simulink library "ifo"  (Simulink 8.2)
settings: Solver=ode45  StartTime=0.0  StopTime=10.0  RelTol=1e-3
undefined symbols (not defined in the file or in its folder): ENUM_EPSADASABREASON_NO_DRIVING_INTERRUPTION, ENUM_GEARPOSN_1ST, ENUM_GEARPOSN_2ND, ENUM_GEARPOSN_3RD, ENUM_GEARPOSN_4TH, ENUM_GEARPOSN_5TH, ENUM_GEARPOSN_6TH, ENUM_LFCSTATE_AUTOSTEERING, ENUM_LFCSTATE_DEGRADED, ENUM_SHIFTLEVER_D, ENUM_SHIFTLEVER_D2, ENUM_SHIFTLEVER_D3, FALSE, KAPP_VehicleWidth_m, KIFO_C1Max4Act_rad, KIFO_C2Max4Act_rat, KIFO_C2Max4Disable_rat, KIFO_C2Max4DisableThr_s, KIFO_DriverStrFightConfirmTime_s, KIFO_DriverStrFightResetTime_s, KIFO_DriverStrFightSetTime_s, KIFO_DriverStrFightThres_Nm, KIFO_DriverStrFightThresHys_Nm, KIFO_DriverStrSoftConfirmTime_s, KIFO_DriverStrSoftResetTime_s, KIFO_DriverStrSoftSetTime_s, KIFO_DriverStrSoftThres_Nm, KIFO_DriverStrStrongConfirmTime_s, KIFO_DriverStrStrongResetTime_s, KIFO_DriverStrStrongSetTime_s, KIFO_DriverStrStrongThres_Nm, KIFO_DriverStrStrongThresHys_Nm, KIFO_Lane4ActThr_s, KIFO_LaneWidthLowThr_m, KIFO_LaneWidthUpThr_m, KIFO_LFCVehSpdMaxLimition_kph, KIFO_LFCVehSpdMimLimition_kph, KIFO_LKAMaxActSpeed_kph, KIFO_LKAMaxDeactSpeed_kph, KIFO_LKAMinActSpeed_kph, KIFO_LKAMinDeactSpeed_kph, KIFO_TLCTriggerThrHysis_s, KIFO_TurnSignalSwOFFTime_s, MIFO_TLCThr4LKA_s, TRUE
libraries: hcu_lib x41, simulink x11, hmi x1, gaps x1, ttc x1, sft x1, veh x1
(part 1 of 2)
settings Model: Creator=xsellart  LastModifiedBy=13192

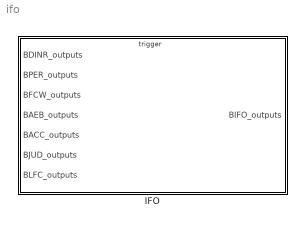
== system ifo ==
  IFO : Subsystem

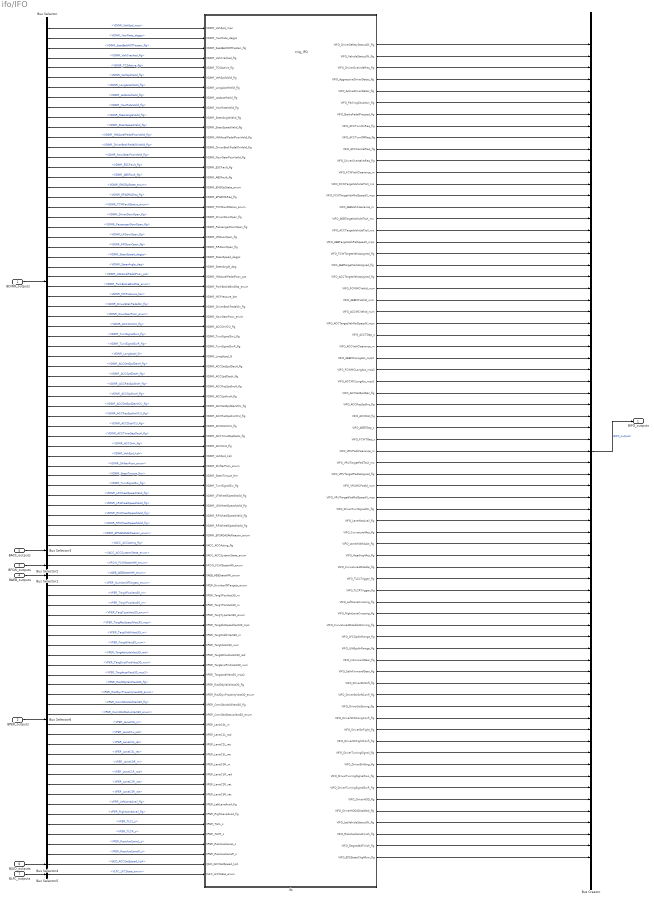
== system ifo/IFO ==
  BDINR_outputs : Inport  OutDataTypeStr=Bus: BDINR_outputs
  BPER_outputs : Inport  Port=2  OutDataTypeStr=Bus: BPER_outputs
  BFCW_outputs : Inport  Port=3  OutDataTypeStr=Bus: BFCW_outputs
  BAEB_outputs : Inport  Port=4  OutDataTypeStr=Bus: BAEB_outputs
  BACC_outputs : Inport  Port=5  OutDataTypeStr=Bus: BACC_outputs
  BJUD_outputs : Inport  Port=6  OutDataTypeStr=Bus: BJUD_outputs
  BLFC_outputs : Inport  Port=7  OutDataTypeStr=Bus: BLFC_outputs
  trig_IFO : TriggerPort  TriggerType=function-call
      settings: AttributesFormatString=State = %<StatesWhenEnabling>
  Bus Creator : BusCreator  Inputs=71  OutDataTypeStr=Bus: BIFO_outputs
  Bus Selector : BusSelector  OutputSignals=VDINR_VehSpd_mps,VDINR_YawRate_degps,VDINR_SeatBeltNOTFasten_flg,VDINR_VehCrashed_flg,VDINR_TCSActive_flg,VDINR_VehSpdValid_flg,VDINR_LongAccelValid_flg,VDINR_LatAccelValid_flg,VDINR_YawRateValid_flg,VDINR_SteerAngleValid_flg,VDINR_SteerSpeedValid_flg,VDINR_HWAccelPedalPosnValid_flg,VDINR_DriverBrakPedalOnValid_flg,VDINR_NowGearPosnValid_flg,VDINR_ESCFault_flg,VDINR_ABSFault_flg,VDINR_EMSOpState_enum,VDINR_EPASMILReq_flg,VDINR_TCMFaultStatus_enum,VDINR_DriverDoorOpen_flg,VDINR_PassengerDoorOpen_flg,VDINR_LRDoorOpen_flg,VDINR_RRDoorOpen_flg,VDINR_SteerSpeed_degps,VDINR_SteerAngle_deg,VDINR_HWAccelPedalPosn_pct,VDINR_ParkBrakeBindSta_enum,VDINR_MCPressure_bar,VDINR_DriverBrakPedalOn_flg,VDINR_NowGearPosn_enum,VDINR_ACCOnVCU_flg,VDINR_TurnSignalSwL_flg,VDINR_TurnSignalSwR_flg,VDINR_LongAccel_G,VDINR_ACCSetSpdDecH_flg,VDINR_ACCSpdDecH_flg,VDINR_ACCResSpdIncH_flg,VDINR_ACCSpdIncH_flg,VDINR_ACCSetSpdDecVCU_flg,VDINR_ACCResSpdIncVCU_flg,VDINR_ACCDistVCU_flg,VDINR_ACCTimeGapDecH_flg,VDINR_ACCOnH_flg,VDINR_VehSpd_kph,VDINR_ShifterPosn_enum,VDINR_SteerTorque_Nm,VDINR_TurnSignalSw_flg,VDINR_LFWheelSpeedValid_flg,VDINR_LRWheelSpeedValid_flg,VDINR_RFWheelSpeedValid_flg,VDINR_RRWheelSpeedValid_flg,VDINR_EPSADASAbReason_enum
  Bus Selector1 : BusSelector  OutputSignals=VAEB_AEBStateHMI_enum
  Bus Selector2 : BusSelector  OutputSignals=VFCW_FCWStateHMI_enum
  Bus Selector3 : BusSelector  OutputSignals=VACC_ACCActing_flg,VACC_ACCSystemState_enum
  Bus Selector4 : BusSelector  OutputSignals=VJUD_ACCSetSpeed_kph
  Bus Selector5 : BusSelector  OutputSignals=VLFC_LFCState_enum
  Bus Selector6 : BusSelector  OutputSignals=VPER_NumberOfTargets_enum,VPER_TargXPosVect30_m,VPER_TargYPosVect30_m,VPER_TargTypeVect30_enum,VPER_TargAbsSpeedVect30_mps,VPER_TargWidthVect30_m,VPER_TargIdVect30_num,VPER_TargAttitudeVect30_rad,VPER_TargExistProbVect30_num,VPER_TargAccelVect30_mps2,VPER_RadObjValidVect30_flg,VPER_RadDynPropertyVect30_enum,VPER_CamObsValidVect30_flg,VPER_CamObsStatusVect30_enum,VPER_LaneC0L_m,VPER_LaneC1L_rad,VPER_LaneC2L_rat,VPER_LaneC3L_rat,VPER_LaneC0R_m,VPER_LaneC1R_rad,VPER_LaneC2R_rat,VPER_LaneC3R_rat,VPER_LeftLaneAvail_flg,VPER_RightLaneAvail_flg,VPER_TLCL_s,VPER_TLCR_s,VPER_ResidualLaneL_s,VPER_ResidualLaneR_s
  ifo : Subsystem
  BIFO_outputs : Outport  OutDataTypeStr=Bus: BIFO_outputs
  wires:
  BDINR_outputs/1 -> Bus Selector/1
  BFCW_outputs/1 -> Bus Selector2/1
  BPER_outputs/1 -> Bus Selector6/1
  Bus Creator/1 -> BIFO_outputs/1  "BIFO_outputs"
  BAEB_outputs/1 -> Bus Selector1/1
  Bus Selector/19 -> ifo/19(VDINR_TCMFaultStatus_enum)  "<VDINR_TCMFaultStatus_enum>"
  Bus Selector/21 -> ifo/21(VDINR_PassengerDoorOpen_flg)  "<VDINR_PassengerDoorOpen_flg>"
  Bus Selector/13 -> ifo/13(VDINR_DriverBrakPedalOnValid_flg)  "<VDINR_DriverBrakPedalOnValid_flg>"
  Bus Selector/11 -> ifo/11(VDINR_SteerSpeedValid_flg)  "<VDINR_SteerSpeedValid_flg>"
  Bus Selector/17 -> ifo/17(VDINR_EMSOpState_enum)  "<VDINR_EMSOpState_enum>"
  Bus Selector/12 -> ifo/12(VDINR_HWAccelPedalPosnValid_flg)  "<VDINR_HWAccelPedalPosnValid_flg>"
  Bus Selector/14 -> ifo/14(VDINR_NowGearPosnValid_flg)  "<VDINR_NowGearPosnValid_flg>"
  Bus Selector/18 -> ifo/18(VDINR_EPASMILReq_flg)  "<VDINR_EPASMILReq_flg>"
  Bus Selector/16 -> ifo/16(VDINR_ABSFault_flg)  "<VDINR_ABSFault_flg>"
  Bus Selector/8 -> ifo/8(VDINR_LatAccelValid_flg)  "<VDINR_LatAccelValid_flg>"
  Bus Selector/20 -> ifo/20(VDINR_DriverDoorOpen_flg)  "<VDINR_DriverDoorOpen_flg>"
  Bus Selector/9 -> ifo/9(VDINR_YawRateValid_flg)  "<VDINR_YawRateValid_flg>"
  Bus Selector/15 -> ifo/15(VDINR_ESCFault_flg)  "<VDINR_ESCFault_flg>"
  Bus Selector/10 -> ifo/10(VDINR_SteerAngleValid_flg)  "<VDINR_SteerAngleValid_flg>"
  Bus Selector/22 -> ifo/22(VDINR_LRDoorOpen_flg)  "<VDINR_LRDoorOpen_flg>"
  Bus Selector/23 -> ifo/23(VDINR_RRDoorOpen_flg)  "<VDINR_RRDoorOpen_flg>"
  Bus Selector/3 -> ifo/3(VDINR_SeatBeltNOTFasten_flg)  "<VDINR_SeatBeltNOTFasten_flg>"
  Bus Selector/6 -> ifo/6(VDINR_VehSpdValid_flg)  "<VDINR_VehSpdValid_flg>"
  Bus Selector/24 -> ifo/24(VDINR_SteerSpeed_degps)  "<VDINR_SteerSpeed_degps>"
  Bus Selector/2 -> ifo/2(VDINR_YawRate_degps)  "<VDINR_YawRate_degps>"
  Bus Selector/4 -> ifo/4(VDINR_VehCrashed_flg)  "<VDINR_VehCrashed_flg>"
  Bus Selector/1 -> ifo/1(VDINR_VehSpd_mps)  "<VDINR_VehSpd_mps>"
  Bus Selector/7 -> ifo/7(VDINR_LongAccelValid_flg)  "<VDINR_LongAccelValid_flg>"
  Bus Selector/5 -> ifo/5(VDINR_TCSActive_flg)  "<VDINR_TCSActive_flg>"
  Bus Selector/30 -> ifo/30(VDINR_NowGearPosn_enum)  "<VDINR_NowGearPosn_enum>"
  Bus Selector/29 -> ifo/29(VDINR_DriverBrakPedalOn_flg)  "<VDINR_DriverBrakPedalOn_flg>"
  Bus Selector/28 -> ifo/28(VDINR_MCPressure_bar)  "<VDINR_MCPressure_bar>"
  Bus Selector/27 -> ifo/27(VDINR_ParkBrakeBindSta_enum)  "<VDINR_ParkBrakeBindSta_enum>"
  Bus Selector/26 -> ifo/26(VDINR_HWAccelPedalPosn_pct)  "<VDINR_HWAccelPedalPosn_pct>"
  Bus Selector/25 -> ifo/25(VDINR_SteerAngle_deg)  "<VDINR_SteerAngle_deg>"
  BACC_outputs/1 -> Bus Selector3/1
  Bus Selector1/1 -> ifo/56(VAEB_AEBStateHMI_enum)  "<VAEB_AEBStateHMI_enum>"
  Bus Selector2/1 -> ifo/55(VFCW_FCWStateHMI_enum)  "<VFCW_FCWStateHMI_enum>"
  Bus Selector3/1 -> ifo/53(VACC_ACCActing_flg)  "<VACC_ACCActing_flg>"
  Bus Selector3/2 -> ifo/54(VACC_ACCSystemState_enum)  "<VACC_ACCSystemState_enum>"
  Bus Selector/32 -> ifo/32(VDINR_TurnSignalSwL_flg)  "<VDINR_TurnSignalSwL_flg>"
  BJUD_outputs/1 -> Bus Selector4/1
  Bus Selector4/1 -> ifo/85(VJUD_ACCSetSpeed_kph)  "<VJUD_ACCSetSpeed_kph>"
  Bus Selector/31 -> ifo/31(VDINR_ACCOnVCU_flg)  "<VDINR_ACCOnVCU_flg>"
  Bus Selector/34 -> ifo/34(VDINR_LongAccel_G)  "<VDINR_LongAccel_G>"
  Bus Selector/35 -> ifo/35(VDINR_ACCSetSpdDecH_flg)  "<VDINR_ACCSetSpdDecH_flg>"
  Bus Selector/36 -> ifo/36(VDINR_ACCSpdDecH_flg)  "<VDINR_ACCSpdDecH_flg>"
  Bus Selector/37 -> ifo/37(VDINR_ACCResSpdIncH_flg)  "<VDINR_ACCResSpdIncH_flg>"
  Bus Selector/38 -> ifo/38(VDINR_ACCSpdIncH_flg)  "<VDINR_ACCSpdIncH_flg>"
  Bus Selector/40 -> ifo/40(VDINR_ACCResSpdIncVCU_flg)  "<VDINR_ACCResSpdIncVCU_flg>"
  Bus Selector/39 -> ifo/39(VDINR_ACCSetSpdDecVCU_flg)  "<VDINR_ACCSetSpdDecVCU_flg>"
  Bus Selector/43 -> ifo/43(VDINR_ACCOnH_flg)  "<VDINR_ACCOnH_flg>"
  Bus Selector/42 -> ifo/42(VDINR_ACCTimeGapDecH_flg)  "<VDINR_ACCTimeGapDecH_flg>"
  Bus Selector/41 -> ifo/41(VDINR_ACCDistVCU_flg)  "<VDINR_ACCDistVCU_flg>"
  Bus Selector/33 -> ifo/33(VDINR_TurnSignalSwR_flg)  "<VDINR_TurnSignalSwR_flg>"
  Bus Selector/44 -> ifo/44(VDINR_VehSpd_kph)  "<VDINR_VehSpd_kph>"
  Bus Selector/45 -> ifo/45(VDINR_ShifterPosn_enum)  "<VDINR_ShifterPosn_enum>"
  Bus Selector/48 -> ifo/48(VDINR_LFWheelSpeedValid_flg)  "<VDINR_LFWheelSpeedValid_flg>"
  Bus Selector/47 -> ifo/47(VDINR_TurnSignalSw_flg)  "<VDINR_TurnSignalSw_flg>"
  Bus Selector/46 -> ifo/46(VDINR_SteerTorque_Nm)  "<VDINR_SteerTorque_Nm>"
  Bus Selector/49 -> ifo/49(VDINR_LRWheelSpeedValid_flg)  "<VDINR_LRWheelSpeedValid_flg>"
  Bus Selector/51 -> ifo/51(VDINR_RRWheelSpeedValid_flg)  "<VDINR_RRWheelSpeedValid_flg>"
  Bus Selector/50 -> ifo/50(VDINR_RFWheelSpeedValid_flg)  "<VDINR_RFWheelSpeedValid_flg>"
  Bus Selector6/8 -> ifo/64(VPER_TargAttitudeVect30_rad)  "<VPER_TargAttitudeVect30_rad>"
  Bus Selector6/9 -> ifo/65(VPER_TargExisProbVect30_num)  "<VPER_TargExistProbVect30_num>"
  Bus Selector6/7 -> ifo/63(VPER_TargIdVect30_num)  "<VPER_TargIdVect30_num>"
  Bus Selector6/6 -> ifo/62(VPER_TargWidthVect30_m)  "<VPER_TargWidthVect30_m>"
  Bus Selector6/10 -> ifo/66(VPER_TargAccelVect30_mps2)  "<VPER_TargAccelVect30_mps2>"
  Bus Selector6/5 -> ifo/61(VPER_TargAbsSpeedVect30_mps)  "<VPER_TargAbsSpeedVect30_mps>"
  Bus Selector6/11 -> ifo/67(VPER_RadObjValidVect30_flg)  "<VPER_RadObjValidVect30_flg>"
  Bus Selector6/4 -> ifo/60(VPER_TargTypeVect30_enum)  "<VPER_TargTypeVect30_enum>"
  Bus Selector6/12 -> ifo/68(VPER_RadDynPropertyVect30_enum)  "<VPER_RadDynPropertyVect30_enum>"
  Bus Selector6/3 -> ifo/59(VPER_TargYPosVect30_m)  "<VPER_TargYPosVect30_m>"
  Bus Selector6/13 -> ifo/69(VPER_CamObsValidVect30_flg)  "<VPER_CamObsValidVect30_flg>"
  Bus Selector6/2 -> ifo/58(VPER_TargXPosVect30_m)  "<VPER_TargXPosVect30_m>"
  Bus Selector6/14 -> ifo/70(VPER_CamObsStatusVect30_enum)  "<VPER_CamObsStatusVect30_enum>"
  Bus Selector6/1 -> ifo/57(VPER_NumberOfTargets_enum)  "<VPER_NumberOfTargets_enum>"
  Bus Selector6/15 -> ifo/71(VPER_LaneC0L_m)  "<VPER_LaneC0L_m>"
  Bus Selector6/16 -> ifo/72(VPER_LaneC1L_rad)  "<VPER_LaneC1L_rad>"
  Bus Selector6/17 -> ifo/73(VPER_LaneC2L_rat)  "<VPER_LaneC2L_rat>"
  Bus Selector6/18 -> ifo/74(VPER_LaneC3L_rat)  "<VPER_LaneC3L_rat>"
  Bus Selector6/19 -> ifo/75(VPER_LaneC0R_m)  "<VPER_LaneC0R_m>"
  Bus Selector6/20 -> ifo/76(VPER_LaneC1R_rad)  "<VPER_LaneC1R_rad>"
  Bus Selector6/21 -> ifo/77(VPER_LaneC2R_rat)  "<VPER_LaneC2R_rat>"
  Bus Selector6/22 -> ifo/78(VPER_LaneC3R_rat)  "<VPER_LaneC3R_rat>"
  Bus Selector6/23 -> ifo/79(VPER_LeftLaneAvail_fig)  "<VPER_LeftLaneAvail_flg>"
  Bus Selector6/24 -> ifo/80(VPER_RightLaneAvail_fig)  "<VPER_RightLaneAvail_flg>"
  Bus Selector6/25 -> ifo/81(VPER_TLCL_s)  "<VPER_TLCL_s>"
  Bus Selector6/26 -> ifo/82(VPER_TLCR_s)  "<VPER_TLCR_s>"
  Bus Selector6/27 -> ifo/83(VPER_ResidualLaneL_s)  "<VPER_ResidualLaneL_s>"
  Bus Selector6/28 -> ifo/84(VPER_ResidualLaneR_s)  "<VPER_ResidualLaneR_s>"
  ifo/17(VIFO_ACCTargetVehicleTtcX_ms) -> Bus Creator/17
  ifo/18(VIFO_AEBTargetVehRelSpeedX_mps) -> Bus Creator/18
  ifo/16(VIFO_AEBTargetVehicleTtcX_ms) -> Bus Creator/16
  ifo/15(VIFO_AEBVehClearance_m) -> Bus Creator/15
  ifo/19(VIFO_FCWTargetVehAssigned_flg) -> Bus Creator/19
  ifo/14(VIFO_FCWTargetVehRelSpeedX_mps) -> Bus Creator/14
  ifo/20(VIFO_AEBTargetVehAssigned_flg) -> Bus Creator/20
  ifo/13(VIFO_FCWTargetVehicleTtcX_ms) -> Bus Creator/13
  ifo/21(VIFO_ACCTargetVehAssigned_flg) -> Bus Creator/21
  ifo/12(VIFO_FCWVehClearance_m) -> Bus Creator/12
  ifo/22(VIFO_FCWMCVehId_num) -> Bus Creator/22
  ifo/11(VIFO_DriverOvertakeReq_flg) -> Bus Creator/11
  ifo/23(VIFO_AEBMCVehId_num) -> Bus Creator/23
  ifo/24(VIFO_ACCMCVehId_num) -> Bus Creator/24
  ifo/10(VIFO_ACCCancelReq_flg) -> Bus Creator/10
  ifo/9(VIFO_ACCTurnOffReq_flg) -> Bus Creator/9
  ifo/25(VIFO_ACCTargetVehRelSpeedX_mps) -> Bus Creator/25
  ifo/8(VIFO_ACCTurnOnReq_flg) -> Bus Creator/8
  ifo/26(VIFO_ACCTGap_s) -> Bus Creator/26
  ifo/7(VIFO_BrakePedalPressed_flg) -> Bus Creator/7
  ifo/27(VIFO_ACCVehClearance_m) -> Bus Creator/27
  ifo/28(VIFO_AEBMCLongAcc_mps2) -> Bus Creator/28
  ifo/6(VIFO_ParkingSituation_flg) -> Bus Creator/6
  ifo/29(VIFO_FCWMCLongAcc_mps2) -> Bus Creator/29
  ifo/5(VIFO_ActiveDriverDetec_flg) -> Bus Creator/5
  ifo/4(VIFO_AggressiveDriverDetec_flg) -> Bus Creator/4
  ifo/30(VIFO_ACCMCLongAcc_mps2) -> Bus Creator/30
  ifo/3(VIFO_DriverOverrideReq_flg) -> Bus Creator/3
  ifo/31(VIFO_ACCSetSpdDec_flg) -> Bus Creator/31
  ifo/32(VIFO_ACCResSpdInc_flg) -> Bus Creator/32
  ifo/2(VIFO_VehicleStatusOk_flg) -> Bus Creator/2
  ifo/1(VIFO_DriverSafetyStatusOk_flg) -> Bus Creator/1
  ifo/33(VIFO_ACCDist_flg) -> Bus Creator/33
  ifo/34(VIFO_AEBTGap_s) -> Bus Creator/34
  ifo/35(VIFO_FCWTGap_s) -> Bus Creator/35
  ifo/36(VIFO_VRUPedClearance_m) -> Bus Creator/36
  ifo/37(VIFO_VRUTargetPedTtcX_ms) -> Bus Creator/37
  ifo/38(VIFO_VRUTargetPedAssigned_flg) -> Bus Creator/38
  ifo/39(VIFO_VRUMCPedId_num) -> Bus Creator/39
  ifo/40(VIFO_VRUTargetPedRelSpeedX_mps) -> Bus Creator/40
  ifo/41(VIFO_DriverTurnSignalOn_flg) -> Bus Creator/41
  ifo/42(VIFO_LaneNotAvail_flg) -> Bus Creator/42
  ifo/43(VIFO_Curvature4Act_flg) -> Bus Creator/43
  ifo/44(VIFO_LaneWidth4Act_flg) -> Bus Creator/44
  ifo/45(VIFO_Heading4Act_flg) -> Bus Creator/45
  ifo/46(VIFO_Curvature4Disable_flg) -> Bus Creator/46
  ifo/47(VIFO_TLCLTrigger_flg) -> Bus Creator/47
  ifo/48(VIFO_TLCRTrigger_flg) -> Bus Creator/48
  ifo/49(VIFO_LeftLaneCrossing_flg) -> Bus Creator/49
  ifo/50(VIFO_RightLaneCrossing_flg) -> Bus Creator/50
  ifo/51(VIFO_Curvature4DisableWarning_flg) -> Bus Creator/51
  ifo/52(VIFO_LFCSpdInRange_flg) -> Bus Creator/52
  ifo/53(VIFO_LKASpdInRange_flg) -> Bus Creator/53
  ifo/54(VIFO_InForwardGear_flg) -> Bus Creator/54
  ifo/55(VIFO_SelInForwardGear_flg) -> Bus Creator/55
  ifo/56(VIFO_DriverStrSoft_flg) -> Bus Creator/56
  ifo/57(VIFO_DriverStrSoftConfi_flg) -> Bus Creator/57
  ifo/58(VIFO_DriverStrStrong_flg) -> Bus Creator/58
  ifo/59(VIFO_DriverStrStrongConfi_flg) -> Bus Creator/59
  ifo/60(VIFO_DriverStrFight_flg) -> Bus Creator/60
  ifo/61(VIFO_DriverStrFightConfi_flg) -> Bus Creator/61
  ifo/62(VIFO_DriverTurningSignal_flg) -> Bus Creator/62
  ifo/63(VIFO_DriverShifting_flg) -> Bus Creator/63
  ifo/64(VIFO_DriverTurningSignalSwL_flg) -> Bus Creator/64
  ifo/65(VIFO_DriverTurningSignalSwR_flg) -> Bus Creator/65
  ifo/66(VIFO_DriverHOD_flg) -> Bus Creator/66
  ifo/67(VIFO_DriverHOD4Disabled_flg) -> Bus Creator/67
  ifo/68(VIFO_LatVehicleStatusOk_flg) -> Bus Creator/68
  ifo/69(VIFO_ResidualLaneFinish_flg) -> Bus Creator/69
  ifo/70(VIFO_DegradedFinish_flg) -> Bus Creator/70
  BLFC_outputs/1 -> Bus Selector5/1
  Bus Selector5/1 -> ifo/86(VLFC_LFCState_enum)  "<VLFC_LFCState_enum>"
  Bus Selector/52 -> ifo/52(VDINR_EPSADASAbReason_enum)  "<VDINR_EPSADASAbReason_enum>"
  ifo/71(VIFO_EPSStateChgAllow_flg) -> Bus Creator/71

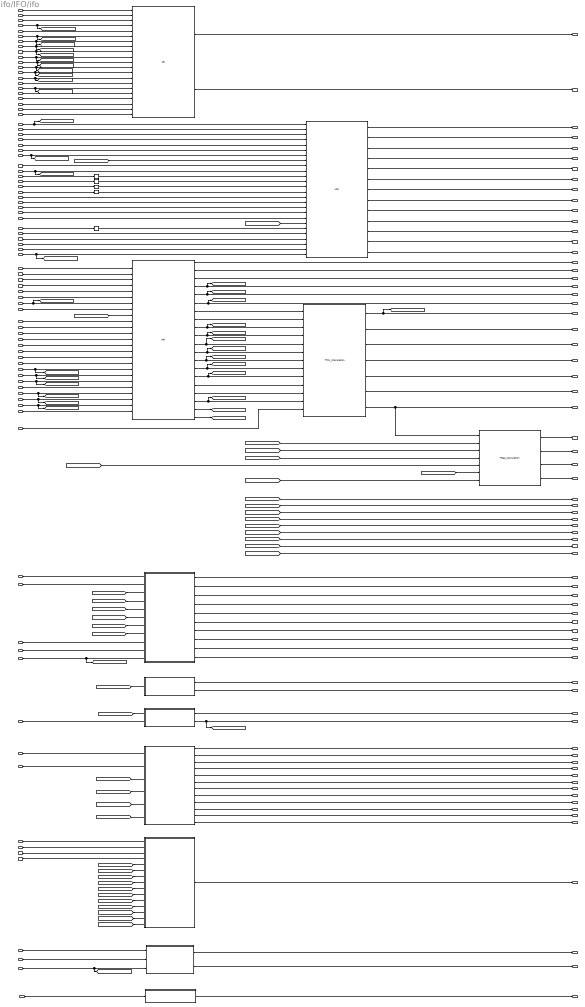
== system ifo/IFO/ifo ==
  VDINR_VehSpd_mps : Inport
  VDINR_YawRate_degps : Inport  Port=2
  VDINR_SeatBeltNOTFasten_flg : Inport  Port=3
  VDINR_VehCrashed_flg : Inport  Port=4
  VDINR_TCSActive_flg : Inport  Port=5
  VDINR_VehSpdValid_flg : Inport  Port=6
  VDINR_LongAccelValid_flg : Inport  Port=7
  VDINR_LatAccelValid_flg : Inport  Port=8
  VDINR_YawRateValid_flg : Inport  Port=9
  VDINR_SteerAngleValid_flg : Inport  Port=10
  VDINR_SteerSpeedValid_flg : Inport  Port=11
  VDINR_HWAccelPedalPosnValid_flg : Inport  Port=12
  VDINR_DriverBrakPedalOnValid_flg : Inport  Port=13
  VDINR_NowGearPosnValid_flg : Inport  Port=14
  VDINR_ESCFault_flg : Inport  Port=15
  VDINR_ABSFault_flg : Inport  Port=16
  VDINR_EMSOpState_enum : Inport  Port=17
  VDINR_EPASMILReq_flg : Inport  Port=18
  VDINR_TCMFaultStatus_enum : Inport  Port=19
  VDINR_DriverDoorOpen_flg : Inport  Port=20
  VDINR_PassengerDoorOpen_flg : Inport  Port=21
  VDINR_LRDoorOpen_flg : Inport  Port=22
  VDINR_RRDoorOpen_flg : Inport  Port=23
  VDINR_SteerSpeed_degps : Inport  Port=24
  VDINR_SteerAngle_deg : Inport  Port=25
  VDINR_HWAccelPedalPosn_pct : Inport  Port=26
  VDINR_ParkBrakeBindSta_enum : Inport  Port=27
  VDINR_MCPressure_bar : Inport  Port=28
  VDINR_DriverBrakPedalOn_flg : Inport  Port=29
  VDINR_NowGearPosn_enum : Inport  Port=30
  VDINR_ACCOnVCU_flg : Inport  Port=31
  VDINR_TurnSignalSwL_flg : Inport  Port=32
  VDINR_TurnSignalSwR_flg : Inport  Port=33
  VDINR_LongAccel_G : Inport  Port=34
  VDINR_ACCSetSpdDecH_flg : Inport  Port=35
  VDINR_ACCSpdDecH_flg : Inport  Port=36
  VDINR_ACCResSpdIncH_flg : Inport  Port=37
  VDINR_ACCSpdIncH_flg : Inport  Port=38
  VDINR_ACCSetSpdDecVCU_flg : Inport  Port=39
  VDINR_ACCResSpdIncVCU_flg : Inport  Port=40
  VDINR_ACCDistVCU_flg : Inport  Port=41
  VDINR_ACCTimeGapDecH_flg : Inport  Port=42
  VDINR_ACCOnH_flg : Inport  Port=43
  VDINR_VehSpd_kph : Inport  Port=44
  VDINR_ShifterPosn_enum : Inport  Port=45
  VDINR_SteerTorque_Nm : Inport  Port=46
  VDINR_TurnSignalSw_flg : Inport  Port=47
  VDINR_LFWheelSpeedValid_flg : Inport  Port=48
  VDINR_LRWheelSpeedValid_flg : Inport  Port=49
  VDINR_RFWheelSpeedValid_flg : Inport  Port=50
  VDINR_RRWheelSpeedValid_flg : Inport  Port=51
  VDINR_EPSADASAbReason_enum : Inport  Port=52
  VACC_ACCActing_flg : Inport  Port=53
  VACC_ACCSystemState_enum : Inport  Port=54
  VFCW_FCWStateHMI_enum : Inport  Port=55
  VAEB_AEBStateHMI_enum : Inport  Port=56
  VPER_NumberOfTargets_enum : Inport  Port=57
  VPER_TargXPosVect30_m : Inport  Port=58
  VPER_TargYPosVect30_m : Inport  Port=59
  VPER_TargTypeVect30_enum : Inport  Port=60
  VPER_TargAbsSpeedVect30_mps : Inport  Port=61
  VPER_TargWidthVect30_m : Inport  Port=62
  VPER_TargIdVect30_num : Inport  Port=63
  VPER_TargAttitudeVect30_rad : Inport  Port=64
  VPER_TargExisProbVect30_num : Inport  Port=65
  VPER_TargAccelVect30_mps2 : Inport  Port=66
  VPER_RadObjValidVect30_flg : Inport  Port=67
  VPER_RadDynPropertyVect30_enum : Inport  Port=68
  VPER_CamObsValidVect30_flg : Inport  Port=69
  VPER_CamObsStatusVect30_enum : Inport  Port=70
  VPER_LaneC0L_m : Inport  Port=71
  VPER_LaneC1L_rad : Inport  Port=72
  VPER_LaneC2L_rat : Inport  Port=73
  VPER_LaneC3L_rat : Inport  Port=74
  VPER_LaneC0R_m : Inport  Port=75
  VPER_LaneC1R_rad : Inport  Port=76
  VPER_LaneC2R_rat : Inport  Port=77
  VPER_LaneC3R_rat : Inport  Port=78
  VPER_LeftLaneAvail_fig : Inport  Port=79
  VPER_RightLaneAvail_fig : Inport  Port=80
  VPER_TLCL_s : Inport  Port=81
  VPER_TLCR_s : Inport  Port=82
  VPER_ResidualLaneL_s : Inport  Port=83
  VPER_ResidualLaneR_s : Inport  Port=84
  VJUD_ACCSetSpeed_kph : Inport  Port=85
  VLFC_LFCState_enum : Inport  Port=86
  Delay{,1..4} (5 alike) : Delay  DelayLength=1  InitialCondition=0
  DriverIntentDecision : Subsystem  TreatAsAtomicUnit=on
  EPSStatus : Subsystem  TreatAsAtomicUnit=on
  HMI : hmi/HMI
  InForwardGearDetection : Subsystem  TreatAsAtomicUnit=on
  LFCLaneWarning_Decision : Subsystem
  LaneInfo : Subsystem  TreatAsAtomicUnit=on
  SpdInRange : Subsystem  TreatAsAtomicUnit=on
  TGap_Calculation : gaps/TGap_Calculation
  TTCx_Calculation : ttc/TTCx_Calculation
  VehicleStatusForLateral : Subsystem  TreatAsAtomicUnit=on
  sft : sft/sft
  veh : veh/veh
  VIFO_DriverSafetyStatusOk_flg : Outport
  VIFO_VehicleStatusOk_flg : Outport  Port=2
  VIFO_DriverOverrideReq_flg : Outport  Port=3
  VIFO_AggressiveDriverDetec_flg : Outport  Port=4
  VIFO_ActiveDriverDetec_flg : Outport  Port=5
  VIFO_ParkingSituation_flg : Outport  Port=6
  VIFO_BrakePedalPressed_flg : Outport  Port=7
  VIFO_ACCTurnOnReq_flg : Outport  Port=8
  VIFO_ACCTurnOffReq_flg : Outport  Port=9
  VIFO_ACCCancelReq_flg : Outport  Port=10
  VIFO_DriverOvertakeReq_flg : Outport  Port=11
  VIFO_FCWVehClearance_m : Outport  Port=12
  VIFO_FCWTargetVehicleTtcX_ms : Outport  Port=13
  VIFO_FCWTargetVehRelSpeedX_mps : Outport  Port=14
  VIFO_AEBVehClearance_m : Outport  Port=15
  VIFO_AEBTargetVehicleTtcX_ms : Outport  Port=16
  VIFO_ACCTargetVehicleTtcX_ms : Outport  Port=17
  VIFO_AEBTargetVehRelSpeedX_mps : Outport  Port=18
  VIFO_FCWTargetVehAssigned_flg : Outport  Port=19
  VIFO_AEBTargetVehAssigned_flg : Outport  Port=20
  VIFO_ACCTargetVehAssigned_flg : Outport  Port=21
  VIFO_FCWMCVehId_num : Outport  Port=22
  VIFO_AEBMCVehId_num : Outport  Port=23
  VIFO_ACCMCVehId_num : Outport  Port=24
  VIFO_ACCTargetVehRelSpeedX_mps : Outport  Port=25
  VIFO_ACCTGap_s : Outport  Port=26
  VIFO_ACCVehClearance_m : Outport  Port=27
  VIFO_AEBMCLongAcc_mps2 : Outport  Port=28
  VIFO_FCWMCLongAcc_mps2 : Outport  Port=29
  VIFO_ACCMCLongAcc_mps2 : Outport  Port=30
  VIFO_ACCSetSpdDec_flg : Outport  Port=31
  VIFO_ACCResSpdInc_flg : Outport  Port=32
  VIFO_ACCDist_flg : Outport  Port=33
  VIFO_AEBTGap_s : Outport  Port=34
  VIFO_FCWTGap_s : Outport  Port=35
  VIFO_VRUPedClearance_m : Outport  Port=36
  VIFO_VRUTargetPedTtcX_ms : Outport  Port=37
  VIFO_VRUTargetPedAssigned_flg : Outport  Port=38
  VIFO_VRUMCPedId_num : Outport  Port=39
  VIFO_VRUTargetPedRelSpeedX_mps : Outport  Port=40
  VIFO_DriverTurnSignalOn_flg : Outport  Port=41
  VIFO_LaneNotAvail_flg : Outport  Port=42
  VIFO_Curvature4Act_flg : Outport  Port=43
  VIFO_LaneWidth4Act_flg : Outport  Port=44
  VIFO_Heading4Act_flg : Outport  Port=45
  VIFO_Curvature4Disable_flg : Outport  Port=46
  VIFO_TLCLTrigger_flg : Outport  Port=47
  VIFO_TLCRTrigger_flg : Outport  Port=48
  VIFO_LeftLaneCrossing_flg : Outport  Port=49
  VIFO_RightLaneCrossing_flg : Outport  Port=50
  VIFO_Curvature4DisableWarning_flg : Outport  Port=51
  VIFO_LFCSpdInRange_flg : Outport  Port=52
  VIFO_LKASpdInRange_flg : Outport  Port=53
  VIFO_InForwardGear_flg : Outport  Port=54
  VIFO_SelInForwardGear_flg : Outport  Port=55
  VIFO_DriverStrSoft_flg : Outport  Port=56
  VIFO_DriverStrSoftConfi_flg : Outport  Port=57
  VIFO_DriverStrStrong_flg : Outport  Port=58
  VIFO_DriverStrStrongConfi_flg : Outport  Port=59
  VIFO_DriverStrFight_flg : Outport  Port=60
  VIFO_DriverStrFightConfi_flg : Outport  Port=61
  VIFO_DriverTurningSignal_flg : Outport  Port=62
  VIFO_DriverShifting_flg : Outport  Port=63
  VIFO_DriverTurningSignalSwL_flg : Outport  Port=64
  VIFO_DriverTurningSignalSwR_flg : Outport  Port=65
  VIFO_DriverHOD_flg : Outport  Port=66
  VIFO_DriverHOD4Disabled_flg : Outport  Port=67
  VIFO_LatVehicleStatusOk_flg : Outport  Port=68
  VIFO_ResidualLaneFinish_flg : Outport  Port=69
  VIFO_DegradedFinish_flg : Outport  Port=70
  VIFO_EPSStateChgAllow_flg : Outport  Port=71
  wires:
  [VIFO_ACCMCLongAcc_mps2] -> VIFO_ACCMCLongAcc_mps2/1
  [VIFO_ACCTargetVehRelSpeedX_mps] -> VIFO_ACCTargetVehRelSpeedX_mps/1
  veh/6 -> [VIFO_ACCTargetVehAssigned_flg], VIFO_ACCTargetVehAssigned_flg/1
  veh/5 -> [VIFO_AEBTargetVehAssigned_flg], VIFO_AEBTargetVehAssigned_flg/1
  veh/4 -> [VIFO_FCWTargetVehAssigned_flg], VIFO_FCWTargetVehAssigned_flg/1
  veh/7 -> TTCx_Calculation/1
  veh/8 -> TTCx_Calculation/2
  veh/9 -> [VIFO_ACCMCVehXPosition_m], TTCx_Calculation/3
  veh/10 -> [VIFO_FCWTargetVehRelSpeedX_mps], TTCx_Calculation/4
  veh/11 -> [VIFO_AEBTargetVehRelSpeedX_mps], TTCx_Calculation/5
  veh/12 -> [VIFO_ACCTargetVehRelSpeedX_mps], TTCx_Calculation/6
  veh/13 -> [VIFO_FCWMCLongAcc_mps2], TTCx_Calculation/7
  veh/14 -> [VIFO_AEBMCLongAcc_mps2], TTCx_Calculation/8
  veh/15 -> [VIFO_ACCMCLongAcc_mps2], TTCx_Calculation/9
  TGap_Calculation/3 -> VIFO_AEBTGap_s/1
  TGap_Calculation/2 -> VIFO_ACCTGap_s/1
  [VDINR_VehSpd_mps] -> TGap_Calculation/5
  [VDINR_VehSpd_mps] -> HMI/8
  HMI/7 -> VIFO_ACCTurnOffReq_flg/1
  veh/2 -> VIFO_AEBMCVehId_num/1
  veh/1 -> VIFO_FCWMCVehId_num/1
  sft/2 -> VIFO_VehicleStatusOk_flg/1
  TTCx_Calculation/2 -> VIFO_FCWTargetVehicleTtcX_ms/1
  sft/1 -> VIFO_DriverSafetyStatusOk_flg/1
  HMI/3 -> VIFO_ActiveDriverDetec_flg/1
  HMI/2 -> VIFO_AggressiveDriverDetec_flg/1
  HMI/4 -> VIFO_ParkingSituation_flg/1
  HMI/5 -> VIFO_BrakePedalPressed_flg/1
  TTCx_Calculation/1 -> VIFO_FCWVehClearance_m/1, [VIFO_FCWVehClearance_m]
  HMI/1 -> VIFO_DriverOverrideReq_flg/1
  TTCx_Calculation/3 -> VIFO_AEBTargetVehicleTtcX_ms/1
  VDINR_SteerAngle_deg/1 -> HMI/1, [VDINR_SteerAngle_deg]
  VDINR_SteerSpeed_degps/1 -> HMI/2
  VDINR_HWAccelPedalPosn_pct/1 -> HMI/3
  VDINR_ParkBrakeBindSta_enum/1 -> HMI/4
  VDINR_DriverBrakPedalOn_flg/1 -> HMI/6
  VDINR_NowGearPosn_enum/1 -> [VDINR_NowGearPosn_enum], HMI/7
  VFCW_FCWStateHMI_enum/1 -> Delay1/1
  VAEB_AEBStateHMI_enum/1 -> Delay/1
  VDINR_EPASMILReq_flg/1 -> [VDINR_EPASMILReq_flg], sft/16
  VDINR_TCMFaultStatus_enum/1 -> sft/17
  VDINR_EMSOpState_enum/1 -> sft/15
  VDINR_ABSFault_flg/1 -> [VDINR_ABSFault_flg], sft/14
  VDINR_DriverDoorOpen_flg/1 -> sft/18
  VDINR_PassengerDoorOpen_flg/1 -> sft/19
  VDINR_ESCFault_flg/1 -> [VDINR_ESCFault_flg], sft/13
  VDINR_LRDoorOpen_flg/1 -> sft/20
  VDINR_NowGearPosnValid_flg/1 -> [VDINR_NowGearPosnValid_flg], sft/12
  VDINR_DriverBrakPedalOnValid_flg/1 -> [VDINR_DriverBrakPedalOnValid_flg], sft/11
  VDINR_RRDoorOpen_flg/1 -> sft/21
  VDINR_SteerSpeedValid_flg/1 -> [VDINR_SteerSpeedValid_flg], sft/9
  VDINR_SteerAngleValid_flg/1 -> [VDINR_SteerAngleValid_flg], sft/8
  VDINR_YawRateValid_flg/1 -> [VDINR_YawRateValid_flg], sft/7
  VDINR_LatAccelValid_flg/1 -> [VDINR_LatAccelValid_flg], sft/6
  VDINR_LongAccelValid_flg/1 -> sft/5
  VDINR_VehSpdValid_flg/1 -> [VDINR_VehSpdValid_flg], sft/4
  VDINR_TCSActive_flg/1 -> sft/3
  VDINR_VehCrashed_flg/1 -> sft/2
  VDINR_SeatBeltNOTFasten_flg/1 -> sft/1
  VDINR_VehSpd_mps/1 -> veh/7, [VDINR_VehSpd_mps]
  VPER_TargAbsSpeedVect30_mps/1 -> veh/5
  VPER_TargTypeVect30_enum/1 -> veh/4
  VPER_TargWidthVect30_m/1 -> veh/6
  VPER_TargXPosVect30_m/1 -> veh/2
  VPER_TargYPosVect30_m/1 -> veh/3
  VDINR_YawRate_degps/1 -> veh/8
  VPER_NumberOfTargets_enum/1 -> veh/1
  [VDINR_SteerAngle_deg] -> veh/9
  VPER_TargIdVect30_num/1 -> veh/10
  VPER_TargAttitudeVect30_rad/1 -> veh/11
  VPER_TargExisProbVect30_num/1 -> veh/12
  [VIFO_AEBTargetVehRelSpeedX_mps] -> VIFO_AEBTargetVehRelSpeedX_mps/1
  [VIFO_FCWTargetVehRelSpeedX_mps] -> VIFO_FCWTargetVehRelSpeedX_mps/1
  VDINR_ACCOnVCU_flg/1 -> HMI/9
  VACC_ACCSystemState_enum/1 -> Delay2/1
  HMI/6 -> VIFO_ACCTurnOnReq_flg/1
  HMI/8 -> VIFO_ACCCancelReq_flg/1
  VACC_ACCActing_flg/1 -> Delay3/1
  TGap_Calculation/1 -> VIFO_ACCVehClearance_m/1
  Delay2/1 -> HMI/13  "VACC_ACCSystemStatePrev_enum"
  Delay/1 -> HMI/12  "VAEB_AEBStateHMIPrev_enum"
  Delay1/1 -> HMI/11  "VFCW_FCWStateHMIPrev_enum"
  VDINR_TurnSignalSwL_flg/1 -> [VDINR_TurnSignalSwL_flg], HMI/10
  HMI/9 -> VIFO_DriverOvertakeReq_flg/1
  [VIFO_ACCTargetVehAssigned_flg] -> HMI/20
  Delay3/1 -> HMI/14  "VACC_ACCActingPrev_flg"
  VDINR_MCPressure_bar/1 -> HMI/5
  VPER_TargAccelVect30_mps2/1 -> veh/13
  VPER_RadObjValidVect30_flg/1 -> veh/14
  VPER_RadDynPropertyVect30_enum/1 -> veh/15
  VPER_CamObsValidVect30_flg/1 -> veh/16
  VPER_CamObsStatusVect30_enum/1 -> veh/17
  VDINR_LongAccel_G/1 -> TTCx_Calculation/13
  veh/3 -> VIFO_ACCMCVehId_num/1
  [VIFO_AEBMCLongAcc_mps2] -> VIFO_AEBMCLongAcc_mps2/1
  [VIFO_FCWMCLongAcc_mps2] -> VIFO_FCWMCLongAcc_mps2/1
  Delay4/1 -> HMI/21  "VJUD_ACCSetSpeedPrev_kph"
  TTCx_Calculation/4 -> VIFO_ACCTargetVehicleTtcX_ms/1
  HMI/10 -> VIFO_ACCSetSpdDec_flg/1
  HMI/11 -> VIFO_ACCResSpdInc_flg/1
  HMI/12 -> VIFO_ACCDist_flg/1
  VDINR_ACCOnH_flg/1 -> HMI/25
  VDINR_ACCTimeGapDecH_flg/1 -> HMI/24
  VDINR_ACCDistVCU_flg/1 -> HMI/23
  VDINR_ACCSetSpdDecH_flg/1 -> HMI/15
  VDINR_ACCSpdDecH_flg/1 -> HMI/16
  VDINR_ACCSetSpdDecVCU_flg/1 -> HMI/17
  VDINR_ACCResSpdIncVCU_flg/1 -> HMI/22
  VDINR_ACCResSpdIncH_flg/1 -> HMI/18
  VDINR_ACCSpdIncH_flg/1 -> HMI/19
  VJUD_ACCSetSpeed_kph/1 -> Delay4/1
  [VIFO_ACCTargetVehAssigned_flg] -> TGap_Calculation/4
  TGap_Calculation/4 -> VIFO_FCWTGap_s/1
  [VIFO_FCWVehClearance_m] -> TGap_Calculation/6
  [VIFO_ACCMCVehXPosition_m] -> TGap_Calculation/3
  [VIFO_FCWTargetVehAssigned_flg] -> TGap_Calculation/7
  TTCx_Calculation/7 -> TGap_Calculation/1, VIFO_AEBVehClearance_m/1
  [VIFO_AEBTargetVehAssigned_flg] -> TGap_Calculation/2
  TTCx_Calculation/5 -> VIFO_VRUPedClearance_m/1
  TTCx_Calculation/6 -> VIFO_VRUTargetPedTtcX_ms/1
  veh/16 -> TTCx_Calculation/10
  veh/17 -> TTCx_Calculation/11
  veh/18 -> [VIFO_VRUTargetPedRelSpeedX_mps], TTCx_Calculation/12
  [VIFO_VRUMCPedId_num] -> VIFO_VRUMCPedId_num/1
  [VIFO_VRUTargetPedAssigned_flg] -> VIFO_VRUTargetPedAssigned_flg/1
  veh/19 -> [VIFO_VRUTargetPedAssigned_flg]
  veh/20 -> [VIFO_VRUMCPedId_num]
  [VIFO_VRUTargetPedRelSpeedX_mps] -> VIFO_VRUTargetPedRelSpeedX_mps/1
  VPER_LaneC0L_m/1 -> [VPER_LaneC0L_m], veh/18
  VPER_LaneC1L_rad/1 -> [VPER_LaneC1L_rad], veh/19
  VPER_LaneC2L_rat/1 -> [VPER_LaneC2L_rat], veh/20
  VPER_LaneC3L_rat/1 -> veh/21
  VPER_LaneC0R_m/1 -> [VPER_LaneC0R_m], veh/22
  VPER_LaneC1R_rad/1 -> [VPER_LaneC1R_rad], veh/23
  VPER_LaneC2R_rat/1 -> [VPER_LaneC2R_rat], veh/24
  VPER_LaneC3R_rat/1 -> veh/25
  VDINR_TurnSignalSwR_flg/1 -> [VDINR_TurnSignalSwR_flg], HMI/26
  HMI/13 -> VIFO_DriverTurnSignalOn_flg/1
  [VPER_LaneC2L_rat] -> LaneInfo/3(VPER_LaneC2L_rat)
  [VPER_LaneC2R_rat] -> LaneInfo/4(VPER_LaneC2R_rat)
  [VPER_LaneC0L_m] -> LaneInfo/5(VPER_LaneC0L_m)
  [VPER_LaneC0R_m] -> LaneInfo/6(VPER_LaneC0R_m)
  [VPER_LaneC1L_rad] -> LaneInfo/7(VPER_LaneC1L_rad)
  [VPER_LaneC1R_rad] -> LaneInfo/8(VPER_LaneC1R_rad)
  VDINR_VehSpd_kph/1 -> [VDINR_VehSpd_kph], LaneInfo/11(VDINR_VehSpd_kph)
  VPER_LeftLaneAvail_fig/1 -> LaneInfo/1("VPER_LeftLaneAvail_fig ")
  VPER_RightLaneAvail_fig/1 -> LaneInfo/2("VPER_RightLaneAvail_fig ")
  VPER_TLCL_s/1 -> LaneInfo/9(VPER_TLCL_s)
  VPER_TLCR_s/1 -> LaneInfo/10(VPER_TLCR_s)
  LaneInfo/1(VIFO_LaneNotAvail_flg) -> VIFO_LaneNotAvail_flg/1
  LaneInfo/2(VIFO_Curvature4Act_flg) -> VIFO_Curvature4Act_flg/1
  LaneInfo/3(VIFO_LaneWidth4Act_flg) -> VIFO_LaneWidth4Act_flg/1
  LaneInfo/4(VIFO_Heading4Act_flg) -> VIFO_Heading4Act_flg/1
  LaneInfo/5(VIFO_Curvature4Disable_flg) -> VIFO_Curvature4Disable_flg/1
  LaneInfo/6(VIFO_TLCLTrigger_flg) -> VIFO_TLCLTrigger_flg/1
  LaneInfo/7(VIFO_TLCRTrigger_flg) -> VIFO_TLCRTrigger_flg/1
  LaneInfo/8(VIFO_LeftLaneCrossing_flg) -> VIFO_LeftLaneCrossing_flg/1
  LaneInfo/9(VIFO_RightLaneCrossing_flg) -> VIFO_RightLaneCrossing_flg/1
  LaneInfo/10(VIFO_Curvature4DisableWarning_flg) -> VIFO_Curvature4DisableWarning_flg/1
  [VDINR_VehSpd_kph] -> SpdInRange/1("VDINR_VehSpd_kph ")
  SpdInRange/1(VIFO_LFCSpdInRange_flg) -> VIFO_LFCSpdInRange_flg/1
  SpdInRange/2(VIFO_LKASpdInRange_flg) -> VIFO_LKASpdInRange_flg/1
  [VDINR_TurnSignalSwR_flg] -> DriverIntentDecision/5(VDINR_TurnSignalSwR_flg)
  [VDINR_TurnSignalSwL_flg] -> DriverIntentDecision/4(VDINR_TurnSignalSwL_flg)
  [VDINR_NowGearPosn_enum] -> InForwardGearDetection/1(VDINR_NowGearPosn_enum)
  InForwardGearDetection/1(VIFO_InForwardGear_flg) -> VIFO_InForwardGear_flg/1
  InForwardGearDetection/2(VIFO_SelInForwardGear_flg) -> [VIFO_SelInForwardGear_flg], VIFO_SelInForwardGear_flg/1
  VDINR_ShifterPosn_enum/1 -> InForwardGearDetection/2(VDINR_ShifterPosn_enum)
  VDINR_SteerTorque_Nm/1 -> DriverIntentDecision/1(VDINR_SteerTorque_Nm)
  VDINR_TurnSignalSw_flg/1 -> DriverIntentDecision/2(VDINR_TurnSignalSw_flg)
  DriverIntentDecision/1(VIFO_DriverStrSoft_flg) -> VIFO_DriverStrSoft_flg/1
  DriverIntentDecision/2(VIFO_DriverStrSoftConfi_flg) -> VIFO_DriverStrSoftConfi_flg/1
  DriverIntentDecision/3(VIFO_DriverStrStrong_flg) -> VIFO_DriverStrStrong_flg/1
  DriverIntentDecision/4(VIFO_DriverStrStrongConfi_flg) -> VIFO_DriverStrStrongConfi_flg/1
  DriverIntentDecision/5(VIFO_DriverStrFight_flg) -> VIFO_DriverStrFight_flg/1
  DriverIntentDecision/6(VIFO_DriverStrFightConfi_flg) -> VIFO_DriverStrFightConfi_flg/1
  DriverIntentDecision/7(VIFO_DriverTurningSignal_flg) -> VIFO_DriverTurningSignal_flg/1
  DriverIntentDecision/8(VIFO_DriverShifting_flg) -> VIFO_DriverShifting_flg/1
  DriverIntentDecision/9(VIFO_DriverTurningSignalSwL_flg) -> VIFO_DriverTurningSignalSwL_flg/1
  DriverIntentDecision/10(VIFO_DriverTurningSignalSwR_flg) -> VIFO_DriverTurningSignalSwR_flg/1
  DriverIntentDecision/11(VIFO_DriverHOD_flg) -> VIFO_DriverHOD_flg/1
  DriverIntentDecision/12(VIFO_DriverHOD4Disabled_flg) -> VIFO_DriverHOD4Disabled_flg/1
  [VIFO_SelInForwardGear_flg] -> DriverIntentDecision/3(VIFO_SelInForwardGear_flg)
  [VDINR_VehSpdValid_flg] -> VehicleStatusForLateral/5(VDINR_VehSpdValid_flg)
  [VDINR_LatAccelValid_flg] -> VehicleStatusForLateral/6(VDINR_LatAccelValid_flg)
  [VDINR_YawRateValid_flg] -> VehicleStatusForLateral/7(VDINR_YawRateValid_flg)
  [VDINR_SteerAngleValid_flg] -> VehicleStatusForLateral/8(VDINR_SteerAngleValid_flg)
  [VDINR_SteerSpeedValid_flg] -> VehicleStatusForLateral/9(VDINR_SteerSpeedValid_flg)
  VDINR_HWAccelPedalPosnValid_flg/1 -> [VDINR_HWAccelPedalPosnValid_flg], sft/10
  [VDINR_HWAccelPedalPosnValid_flg] -> VehicleStatusForLateral/10(VDINR_HWAccelPedalPosnValid_flg)
  [VDINR_DriverBrakPedalOnValid_flg] -> VehicleStatusForLateral/11(VDINR_DriverBrakPedalOnValid_flg)
  [VDINR_NowGearPosnValid_flg] -> VehicleStatusForLateral/12(VDINR_NowGearPosnValid_flg)
  [VDINR_ESCFault_flg] -> VehicleStatusForLateral/13(VDINR_ESCFault_flg)
  [VDINR_ABSFault_flg] -> VehicleStatusForLateral/14(VDINR_ABSFault_flg)
  [VDINR_EPASMILReq_flg] -> VehicleStatusForLateral/15(VDINR_EPASMILReq_flg)
  VehicleStatusForLateral/1(VIFO_LatVehicleStatusOk_flg) -> VIFO_LatVehicleStatusOk_flg/1
  VDINR_LFWheelSpeedValid_flg/1 -> VehicleStatusForLateral/1(VDINR_LFWheelSpeedValid_flg)
  VDINR_RFWheelSpeedValid_flg/1 -> VehicleStatusForLateral/3(VDINR_RFWheelSpeedValid_flg)
  VDINR_LRWheelSpeedValid_flg/1 -> VehicleStatusForLateral/2(VDINR_LRWheelSpeedValid_flg)
  VDINR_RRWheelSpeedValid_flg/1 -> VehicleStatusForLateral/4(VDINR_RRWheelSpeedValid_flg)
  VPER_ResidualLaneL_s/1 -> LFCLaneWarning_Decision/1(VPER_ResidualLaneL_s)
  VPER_ResidualLaneR_s/1 -> LFCLaneWarning_Decision/2(VPER_ResidualLaneR_s)
  LFCLaneWarning_Decision/1(VIFO_ResidualLaneFinish_flg) -> VIFO_ResidualLaneFinish_flg/1
  LFCLaneWarning_Decision/2(VIFO_DegradedFinish_flg) -> VIFO_DegradedFinish_flg/1
  VLFC_LFCState_enum/1 -> [VLFC_LFCState_enum], LFCLaneWarning_Decision/3(VLFC_LFCState_enum)
  [VLFC_LFCState_enum] -> DriverIntentDecision/6(VLFC_LFCState_enum)
  VDINR_EPSADASAbReason_enum/1 -> EPSStatus/1(VDINR_EPSADASAbReason_enum)
  EPSStatus/1(VIFO_EPSStateChgAllow_flg) -> VIFO_EPSStateChgAllow_flg/1

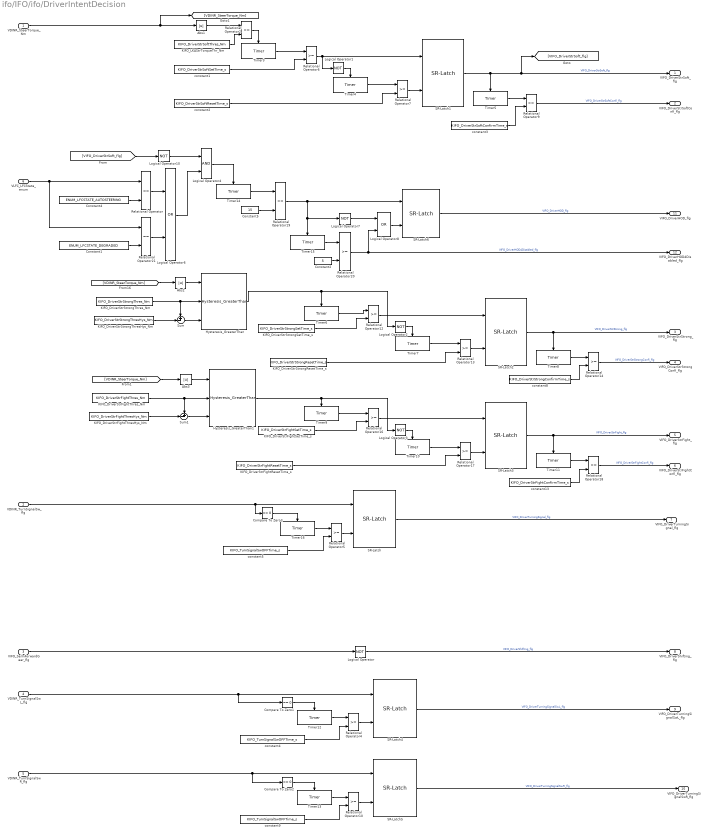
== system ifo/IFO/ifo/DriverIntentDecision ==
  VDINR_SteerTorque_Nm : Inport
  VDINR_TurnSignalSw_flg : Inport  Port=2
  VIFO_SelInForwardGear_flg : Inport  Port=3
  VDINR_TurnSignalSwL_flg : Inport  Port=4
  VDINR_TurnSignalSwR_flg : Inport  Port=5
  VLFC_LFCState_enum : Inport  Port=6
  Abs1 : Abs
  Abs2 : Abs
  Abs3 : Abs
  Compare To Zero1 : simulink/Logic and Bit Operations/Compare To Zero  relop===  OutDataTypeStr=uint8  ZeroCross=off
  Compare To Zero2 : simulink/Logic and Bit Operations/Compare To Zero  relop===  OutDataTypeStr=uint8  ZeroCross=off
  Compare To Zero3 : simulink/Logic and Bit Operations/Compare To Zero  relop===  OutDataTypeStr=uint8  ZeroCross=off
  Constant1 : Constant  Value=ENUM_LFCSTATE_DEGRADED
  Constant2 : Constant  Value=5  OutDataTypeStr=single
  Constant4 : Constant  Value=ENUM_LFCSTATE_AUTOSTEERING
  Constant5 : Constant  Value=15  OutDataTypeStr=single
  Hysteresis_GreaterThan : hcu_lib/Hysteresis_GreaterThan  SystemSampleTime=-1
  Hysteresis_GreaterThan1 : hcu_lib/Hysteresis_GreaterThan  SystemSampleTime=-1
  KIFO_DriverStrFightResetTime_s : Constant  Value=KIFO_DriverStrFightResetTime_s
  KIFO_DriverStrFightSetTime_s : Constant  Value=KIFO_DriverStrFightSetTime_s
  KIFO_DriverStrFightThresHys_Nm : Constant  Value=KIFO_DriverStrFightThresHys_Nm
  KIFO_DriverStrFightThres_Nm : Constant  Value=KIFO_DriverStrFightThres_Nm
  KIFO_DriverStrStrongResetTime_s : Constant  Value=KIFO_DriverStrStrongResetTime_s
  KIFO_DriverStrStrongSetTime_s : Constant  Value=KIFO_DriverStrStrongSetTime_s
  KIFO_DriverStrStrongThresHys_Nm : Constant  Value=KIFO_DriverStrStrongThresHys_Nm
  KIFO_DriverStrStrongThres_Nm : Constant  Value=KIFO_DriverStrStrongThres_Nm
  KIFO_LKAStrTorqueThr_Nm : Constant  Value=KIFO_DriverStrSoftThres_Nm
  Logical Operator{,1..3,7,10} (6 alike) : Logic  Operator=NOT  AllPortsSameDT=off  OutDataTypeStr=boolean
  Logical Operator4 : Logic  AllPortsSameDT=off  OutDataTypeStr=boolean
  Logical Operator6 : Logic  Operator=OR  AllPortsSameDT=off  OutDataTypeStr=boolean
  Logical Operator8 : Logic  Operator=OR  AllPortsSameDT=off  OutDataTypeStr=boolean
  Relational Operator : RelationalOperator  Operator===  OutDataTypeStr=boolean
  Relational Operator{2,4..7,9..10,12..14,16..20} (15 alike) : RelationalOperator  OutDataTypeStr=boolean
  Relational Operator21 : RelationalOperator  Operator===  OutDataTypeStr=boolean
  SR-Latch{,1..6} (7 alike) : hcu_lib/SR-Latch  SystemSampleTime=-1
  Sum : Sum  Inputs=+-|
  Sum1 : Sum  Inputs=+-|
  Timer{3..16} (14 alike) : hcu_lib/Timer  SystemSampleTime=-1
  constant1 : Constant  Value=KIFO_DriverStrSoftSetTime_s
  constant13 : Constant  Value=KIFO_DriverStrFightConfirmTime_s
  constant2 : Constant  Value=KIFO_DriverStrSoftResetTime_s
  constant3 : Constant  Value=KIFO_DriverStrSoftConfirmTime_s
  constant4 : Constant  Value=KIFO_TurnSignalSwOFFTime_s
  constant5 : Constant  Value=KIFO_TurnSignalSwOFFTime_s
  constant8 : Constant  Value=KIFO_DriverStrStrongConfirmTime_s
  constant9 : Constant  Value=KIFO_TurnSignalSwOFFTime_s
  VIFO_DriverStrSoft_flg : Outport
  VIFO_DriverStrSoftConfi_flg : Outport  Port=2
  VIFO_DriverStrStrong_flg : Outport  Port=3
  VIFO_DriverStrStrongConfi_flg : Outport  Port=4
  VIFO_DriverStrFight_flg : Outport  Port=5
  VIFO_DriverStrFightConfi_flg : Outport  Port=6
  VIFO_DriverTurningSignal_flg : Outport  Port=7
  VIFO_DriverShifting_flg : Outport  Port=8
  VIFO_DriverTurningSignalSwL_flg : Outport  Port=9
  VIFO_DriverTurningSignalSwR_flg : Outport  Port=10
  VIFO_DriverHOD_flg : Outport  Port=11
  VIFO_DriverHOD4Disabled_flg : Outport  Port=12
  wires:
  VIFO_SelInForwardGear_flg/1 -> Logical Operator/1
  VDINR_TurnSignalSw_flg/1 -> Compare To Zero3/1, SR-Latch/1
  Logical Operator/1 -> VIFO_DriverShifting_flg/1  "VIFO_DriverShifting_flg"
  SR-Latch/1 -> VIFO_DriverTurningSignal_flg/1  "VIFO_DriverTurningSignal_flg"
  KIFO_LKAStrTorqueThr_Nm/1 -> Relational Operator2/2
  VDINR_SteerTorque_Nm/1 -> [VDINR_SteerTorque_Nm], Abs1/1
  Abs1/1 -> Relational Operator2/1
  Relational Operator2/1 -> Timer3/Enable
  Timer3/1 -> Relational Operator6/1
  constant1/1 -> Relational Operator6/2
  Relational Operator6/1 -> Logical Operator1/1, SR-Latch1/1
  Logical Operator1/1 -> Timer4/Enable
  constant2/1 -> Relational Operator7/2
  Timer4/1 -> Relational Operator7/1
  Relational Operator7/1 -> SR-Latch1/2
  SR-Latch1/1 -> [VIFO_DriverStrSoft_flg], VIFO_DriverStrSoft_flg/1, Timer5/Enable  "VIFO_DriverStrSoft_flg"
  Timer5/1 -> Relational Operator9/1
  constant3/1 -> Relational Operator9/2
  Relational Operator9/1 -> VIFO_DriverStrSoftConfi_flg/1  "VIFO_DriverStrSoftConfi_flg"
  KIFO_DriverStrStrongThres_Nm/1 -> Sum/1, Hysteresis_GreaterThan/2
  [VDINR_SteerTorque_Nm] -> Abs2/1
  Abs2/1 -> Hysteresis_GreaterThan/1
  Timer6/1 -> Relational Operator12/1
  KIFO_DriverStrStrongSetTime_s/1 -> Relational Operator12/2
  Relational Operator12/1 -> SR-Latch2/1
  Logical Operator2/1 -> Timer7/Enable
  KIFO_DriverStrStrongResetTime_s/1 -> Relational Operator13/2
  Timer7/1 -> Relational Operator13/1
  Relational Operator13/1 -> SR-Latch2/2
  SR-Latch2/1 -> VIFO_DriverStrStrong_flg/1, Timer8/Enable  "VIFO_DriverStrStrong_flg"
  Timer8/1 -> Relational Operator14/1
  constant8/1 -> Relational Operator14/2
  Relational Operator14/1 -> VIFO_DriverStrStrongConfi_flg/1  "VIFO_DriverStrStrongConfi_flg"
  KIFO_DriverStrFightThres_Nm/1 -> Sum1/1, Hysteresis_GreaterThan1/2
  [VDINR_SteerTorque_Nm] -> Abs3/1
  Abs3/1 -> Hysteresis_GreaterThan1/1
  Hysteresis_GreaterThan1/1 -> Logical Operator3/1, Timer9/Enable
  Timer9/1 -> Relational Operator16/1
  KIFO_DriverStrFightSetTime_s/1 -> Relational Operator16/2
  Relational Operator16/1 -> SR-Latch3/1
  Logical Operator3/1 -> Timer10/Enable
  KIFO_DriverStrFightResetTime_s/1 -> Relational Operator17/2
  Timer10/1 -> Relational Operator17/1
  Relational Operator17/1 -> SR-Latch3/2
  SR-Latch3/1 -> VIFO_DriverStrFight_flg/1, Timer11/Enable  "VIFO_DriverStrFight_flg"
  Timer11/1 -> Relational Operator18/1
  constant13/1 -> Relational Operator18/2
  Relational Operator18/1 -> VIFO_DriverStrFightConfi_flg/1  "VIFO_DriverStrFightConfi_flg"
  Sum/1 -> Hysteresis_GreaterThan/3
  KIFO_DriverStrStrongThresHys_Nm/1 -> Sum/2
  Hysteresis_GreaterThan/1 -> Timer6/Enable, Logical Operator2/1
  Sum1/1 -> Hysteresis_GreaterThan1/3
  KIFO_DriverStrFightThresHys_Nm/1 -> Sum1/2
  VDINR_TurnSignalSwL_flg/1 -> Compare To Zero1/1, SR-Latch4/1
  Compare To Zero1/1 -> Timer12/Enable
  Timer12/1 -> Relational Operator4/1
  Relational Operator4/1 -> SR-Latch4/2
  constant4/1 -> Relational Operator4/2
  SR-Latch4/1 -> VIFO_DriverTurningSignalSwL_flg/1  "VIFO_DriverTurningSignalSwL_flg"
  Compare To Zero2/1 -> Timer13/Enable
  Timer13/1 -> Relational Operator10/1
  Relational Operator10/1 -> SR-Latch5/2
  constant9/1 -> Relational Operator10/2
  SR-Latch5/1 -> VIFO_DriverTurningSignalSwR_flg/1  "VIFO_DriverTurningSignalSwR_flg"
  VDINR_TurnSignalSwR_flg/1 -> Compare To Zero2/1, SR-Latch5/1
  Logical Operator10/1 -> Logical Operator4/1
  Timer14/1 -> Relational Operator19/1
  Constant5/1 -> Relational Operator19/2
  Logical Operator8/1 -> SR-Latch6/2
  SR-Latch6/1 -> VIFO_DriverHOD_flg/1  "VIFO_DriverHOD_flg"
  [VIFO_DriverStrSoft_flg] -> Logical Operator10/1
  Relational Operator20/1 -> VIFO_DriverHOD4Disabled_flg/1, Logical Operator8/2  "VIFO_DriverHOD4Disabled_flg"
  Logical Operator7/1 -> Logical Operator8/1
  Timer15/1 -> Relational Operator20/1
  Relational Operator19/1 -> Logical Operator7/1, Timer15/Enable, SR-Latch6/1
  Constant2/1 -> Relational Operator20/2
  Logical Operator4/1 -> Timer14/Enable
  VLFC_LFCState_enum/1 -> Relational Operator21/1, Relational Operator/1
  Constant4/1 -> Relational Operator/2
  Constant1/1 -> Relational Operator21/2
  Relational Operator/1 -> Logical Operator6/1
  Relational Operator21/1 -> Logical Operator6/2
  Logical Operator6/1 -> Logical Operator4/2
  Compare To Zero3/1 -> Timer16/Enable
  Timer16/1 -> Relational Operator5/1
  constant5/1 -> Relational Operator5/2
  Relational Operator5/1 -> SR-Latch/2

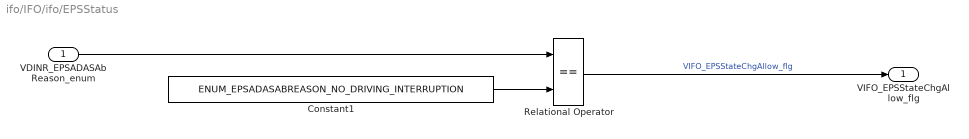
== system ifo/IFO/ifo/EPSStatus ==
  VDINR_EPSADASAbReason_enum : Inport
  Constant1 : Constant  Value=ENUM_EPSADASABREASON_NO_DRIVING_INTERRUPTION
  Relational Operator : RelationalOperator  Operator===  OutDataTypeStr=boolean
  VIFO_EPSStateChgAllow_flg : Outport
  wires:
  VDINR_EPSADASAbReason_enum/1 -> Relational Operator/1
  Constant1/1 -> Relational Operator/2
  Relational Operator/1 -> VIFO_EPSStateChgAllow_flg/1  "VIFO_EPSStateChgAllow_flg"

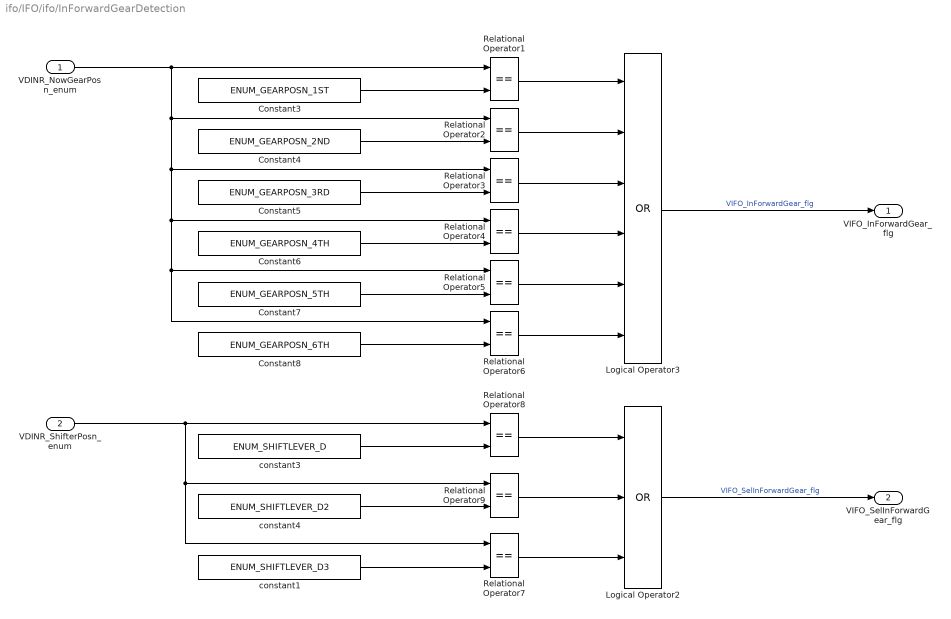
== system ifo/IFO/ifo/InForwardGearDetection ==
  VDINR_NowGearPosn_enum : Inport
  VDINR_ShifterPosn_enum : Inport  Port=2
  Constant3 : Constant  Value=ENUM_GEARPOSN_1ST
  Constant4 : Constant  Value=ENUM_GEARPOSN_2ND
  Constant5 : Constant  Value=ENUM_GEARPOSN_3RD
  Constant6 : Constant  Value=ENUM_GEARPOSN_4TH
  Constant7 : Constant  Value=ENUM_GEARPOSN_5TH
  Constant8 : Constant  Value=ENUM_GEARPOSN_6TH
  Logical Operator2 : Logic  Operator=OR  Inputs=3  AllPortsSameDT=off  OutDataTypeStr=boolean
  Logical Operator3 : Logic  Operator=OR  Inputs=6  AllPortsSameDT=off  OutDataTypeStr=boolean
  Relational Operator{1..9} (9 alike) : RelationalOperator  Operator===  OutDataTypeStr=boolean
  constant1 : Constant  Value=ENUM_SHIFTLEVER_D3
  constant3 : Constant  Value=ENUM_SHIFTLEVER_D
  constant4 : Constant  Value=ENUM_SHIFTLEVER_D2
  VIFO_InForwardGear_flg : Outport
  VIFO_SelInForwardGear_flg : Outport  Port=2
  wires:
  Relational Operator1/1 -> Logical Operator3/1
  Logical Operator3/1 -> VIFO_InForwardGear_flg/1  "VIFO_InForwardGear_flg"
  Constant6/1 -> Relational Operator4/2
  Constant4/1 -> Relational Operator2/2
  VDINR_NowGearPosn_enum/1 -> Relational Operator1/1, Relational Operator6/1, Relational Operator5/1, Relational Operator4/1, Relational Operator3/1, Relational Operator2/1
  Relational Operator5/1 -> Logical Operator3/5
  Constant3/1 -> Relational Operator1/2
  Relational Operator2/1 -> Logical Operator3/2
  Relational Operator6/1 -> Logical Operator3/6
  Constant5/1 -> Relational Operator3/2
  Relational Operator4/1 -> Logical Operator3/4
  Constant7/1 -> Relational Operator5/2
  Relational Operator3/1 -> Logical Operator3/3
  Constant8/1 -> Relational Operator6/2
  Logical Operator2/1 -> VIFO_SelInForwardGear_flg/1  "VIFO_SelInForwardGear_flg"
  VDINR_ShifterPosn_enum/1 -> Relational Operator9/1, Relational Operator7/1, Relational Operator8/1
  Relational Operator8/1 -> Logical Operator2/1
  constant3/1 -> Relational Operator8/2
  constant4/1 -> Relational Operator9/2
  constant1/1 -> Relational Operator7/2
  Relational Operator9/1 -> Logical Operator2/2
  Relational Operator7/1 -> Logical Operator2/3

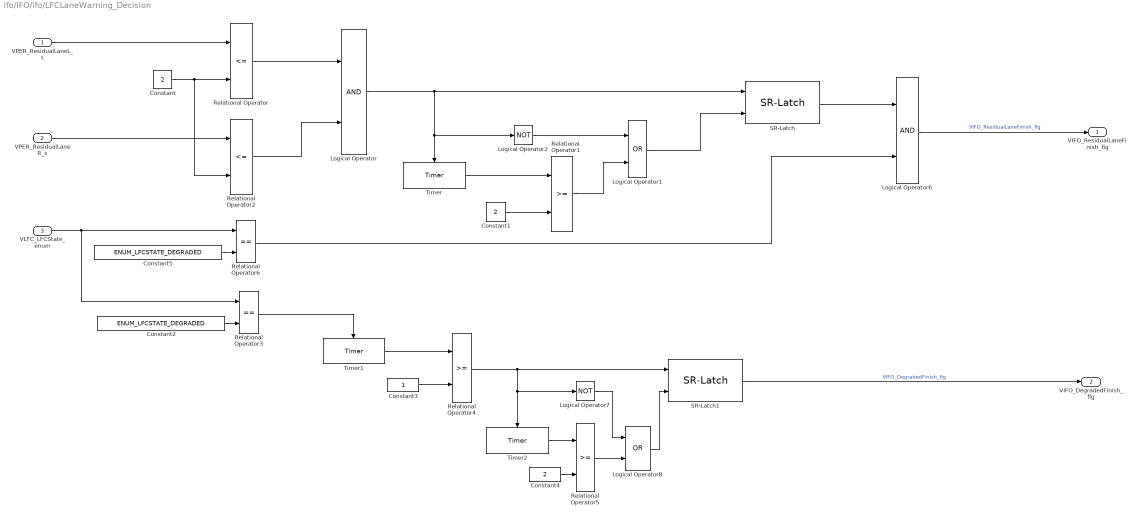
== system ifo/IFO/ifo/LFCLaneWarning_Decision ==
  VPER_ResidualLaneL_s : Inport
  VPER_ResidualLaneR_s : Inport  Port=2
  VLFC_LFCState_enum : Inport  Port=3
  Constant : Constant  Value=2  OutDataTypeStr=single
  Constant1 : Constant  Value=2  OutDataTypeStr=single
  Constant2 : Constant  Value=ENUM_LFCSTATE_DEGRADED
  Constant3 : Constant  OutDataTypeStr=single
  Constant4 : Constant  Value=2  OutDataTypeStr=single
  Constant5 : Constant  Value=ENUM_LFCSTATE_DEGRADED
  Logical Operator : Logic  AllPortsSameDT=off  OutDataTypeStr=boolean
  Logical Operator1 : Logic  Operator=OR  AllPortsSameDT=off  OutDataTypeStr=boolean
  Logical Operator2 : Logic  Operator=NOT  AllPortsSameDT=off  OutDataTypeStr=boolean
  Logical Operator6 : Logic  AllPortsSameDT=off  OutDataTypeStr=boolean
  Logical Operator7 : Logic  Operator=NOT  AllPortsSameDT=off  OutDataTypeStr=boolean
  Logical Operator8 : Logic  Operator=OR  AllPortsSameDT=off  OutDataTypeStr=boolean
  Relational Operator : RelationalOperator  Operator=<=  OutDataTypeStr=boolean
  Relational Operator1 : RelationalOperator  OutDataTypeStr=boolean
  Relational Operator2 : RelationalOperator  Operator=<=  OutDataTypeStr=boolean
  Relational Operator3 : RelationalOperator  Operator===  OutDataTypeStr=boolean
  Relational Operator4 : RelationalOperator  OutDataTypeStr=boolean
  Relational Operator5 : RelationalOperator  OutDataTypeStr=boolean
  Relational Operator6 : RelationalOperator  Operator===  OutDataTypeStr=boolean
  SR-Latch : hcu_lib/SR-Latch  SystemSampleTime=-1
  SR-Latch1 : hcu_lib/SR-Latch  SystemSampleTime=-1
  Timer : hcu_lib/Timer  SystemSampleTime=-1
  Timer1 : hcu_lib/Timer  SystemSampleTime=-1
  Timer2 : hcu_lib/Timer  SystemSampleTime=-1
  VIFO_ResidualLaneFinish_flg : Outport
  VIFO_DegradedFinish_flg : Outport  Port=2
  wires:
  Relational Operator/1 -> Logical Operator/1
  Relational Operator2/1 -> Logical Operator/2
  Timer/1 -> Relational Operator1/1
  Logical Operator1/1 -> SR-Latch/2
  VPER_ResidualLaneL_s/1 -> Relational Operator/1
  Constant/1 -> Relational Operator2/2, Relational Operator/2
  Logical Operator2/1 -> Logical Operator1/1
  VPER_ResidualLaneR_s/1 -> Relational Operator2/1
  Logical Operator/1 -> Logical Operator2/1, Timer/Enable, SR-Latch/1
  Relational Operator1/1 -> Logical Operator1/2
  Constant1/1 -> Relational Operator1/2
  Logical Operator6/1 -> VIFO_ResidualLaneFinish_flg/1  "VIFO_ResidualLaneFinish_flg"
  Relational Operator3/1 -> Timer1/Enable
  Relational Operator5/1 -> Logical Operator8/2
  Logical Operator7/1 -> Logical Operator8/1
  Timer2/1 -> Relational Operator5/1
  Logical Operator8/1 -> SR-Latch1/2
  Timer1/1 -> Relational Operator4/1
  Relational Operator4/1 -> SR-Latch1/1, Logical Operator7/1, Timer2/Enable
  Constant3/1 -> Relational Operator4/2
  Constant4/1 -> Relational Operator5/2
  Constant2/1 -> Relational Operator3/2
  SR-Latch/1 -> Logical Operator6/1
  Constant5/1 -> Relational Operator6/2
  VLFC_LFCState_enum/1 -> Relational Operator3/1, Relational Operator6/1
  Relational Operator6/1 -> Logical Operator6/2
  SR-Latch1/1 -> VIFO_DegradedFinish_flg/1  "VIFO_DegradedFinish_flg"
